simulink model "Der_Faux_FPGA_V2_optimized_synthesizable"  (R2020a)
settings: Solver=FixedStepDiscrete  StartTime=0.0  StopTime=0.84375  FixedStep=1/fs_sim  RelTol=1e-3
values from neighbouring files (symbols this model uses):
  ADC_res = 5    [Der_Faux_ctr_FPGA.m]
  ADC_res_G4 = 8    [Der_Faux_ctr_FPGA.m]
  fs = 48000    [Der_Faux_ctr_FPGA.m]
  fs_sim = fs*ovs    (= 6144000)    [Der_Faux_ctr_FPGA.m]
  Gvar1_N = fi(Gvar1_N,0,ADC_res,0)    [Der_Faux_ctr_FPGA.m]
  Gvar2_N = fi(Gvar2_N,0,ADC_res,0)    [Der_Faux_ctr_FPGA.m]
  Gvar3_N = fi(Gvar3_N,0,ADC_res,0)    [Der_Faux_ctr_FPGA.m]
  Gvar4_N = fi(Gvar4_N,0,ADC_res_G4,0)    [Der_Faux_ctr_FPGA.m]
  input_space = linspace(0,2^ADC_res-1,2^ADC_res)    [Der_Faux_ctr_FPGA.m]
  input_spcae_extended = linspace(0,(2^ADC_res)^3-1,(2^ADC_res)^3)    [Der_Faux_ctr_FPGA.m]
  LUT_Z22a_opt = sfi(LUT_Z22a, len_LUT22a)    [Der_Faux_ctr_FPGA.m]
  LUT_Z22b_opt = sfi(LUT_Z22b, len_LUT22b)    [Der_Faux_ctr_FPGA.m]
  LUT_Z23a_opt = sfi(LUT_Z23a, len_Z23a)    [Der_Faux_ctr_FPGA.m]
  LUT_Z23b_opt = sfi(LUT_Z23b, len_Z23b)    [Der_Faux_ctr_FPGA.m]
  LUT_Z24a_opt = sfi(LUT_Z24a, len_LUT24a)    [Der_Faux_ctr_FPGA.m]
  LUT_Z24b_opt = sfi(LUT_Z24b, len_LUT24b)    [Der_Faux_ctr_FPGA.m]
  LUT_Z25a_opt = sfi(LUT_Z25a, len_LUT25a)    [Der_Faux_ctr_FPGA.m]
  LUT_Z25b_opt = sfi(LUT_Z25b, len_LUT25b)    [Der_Faux_ctr_FPGA.m]
  shift_reg_size = 8*44000    (= 352000)    [Der_Faux_ctr_FPGA.m]
  use_stimuli = [true,true,true,true]    [Der_Faux_ctr_FPGA.m]
  WL_RAM = 5    [Der_Faux_ctr_FPGA.m]
undefined symbols (not defined in the file or in its folder): poti_stimuli1, poti_stimuli2, poti_stimuli3, poti_stimuli4
libraries: hdlmdlgenlib x30, simulink x6, hdlsllib x4
(part 3 of 3)

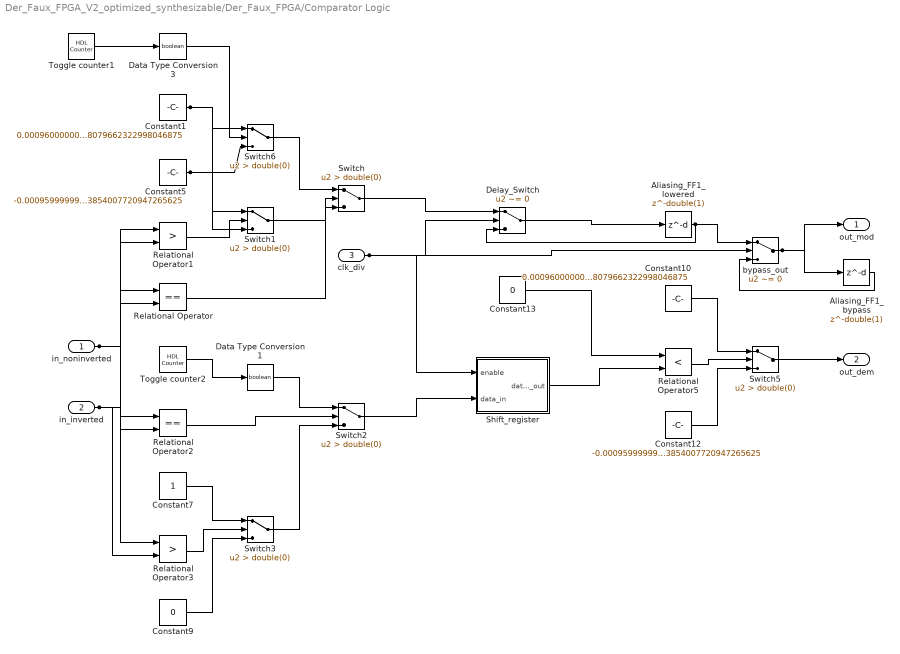
== system Der_Faux_FPGA_V2_optimized_synthesizable/Der_Faux_FPGA/Comparator Logic ==
  in_noninverted : Inport  OutDataTypeStr=fixdt(1, 46, 42)  PortDimensions=1  SampleTime=1.62760416666667e-07
  in_inverted : Inport  Port=2  OutDataTypeStr=fixdt(1, 46, 42)  PortDimensions=1  SampleTime=1.62760416666667e-07
  clk_div : Inport  Port=3  OutDataTypeStr=boolean  PortDimensions=1  SampleTime=1.62760416666667e-07  LockScale=on
  Aliasing_FF1_bypass : Delay  DelayLength=double(1)  SampleTime=1.62760416666667e-07
  Aliasing_FF1_lowered : Delay  DelayLength=double(1)  InitialCondition=0  SampleTime=1.62760416666667e-07
  Constant1 : Constant  Value=0.00096000000000000251798581984985503368079662322998046875  OutDataTypeStr=fixdt(0, 46, 56)  SampleTime=1.62760416666667e-07
  Constant10 : Constant  Value=0.00096000000000000251798581984985503368079662322998046875  OutDataTypeStr=fixdt(0, 46, 56)  SampleTime=1.62760416666667e-07
  Constant12 : Constant  Value=-0.0009599999999999886401980120353982783854007720947265625  OutDataTypeStr=fixdt(1, 46, 55)  SampleTime=1.62760416666667e-07
  Constant13 : Constant  Value=0  OutDataTypeStr=boolean  SampleTime=1.62760416666667e-07
  Constant5 : Constant  Value=-0.0009599999999999886401980120353982783854007720947265625  OutDataTypeStr=fixdt(1, 46, 55)  SampleTime=1.62760416666667e-07
  Constant7 : Constant  OutDataTypeStr=boolean  SampleTime=1.62760416666667e-07
  Constant9 : Constant  Value=0  OutDataTypeStr=boolean  SampleTime=1.62760416666667e-07
  Data Type Conversion1 : DataTypeConversion  OutDataTypeStr=boolean  SampleTime=1.62760416666667e-07
  Data Type Conversion3 : DataTypeConversion  OutDataTypeStr=boolean  SampleTime=1.62760416666667e-07
  Delay_Switch : Switch  Criteria=u2 ~= 0  Threshold=double(0)  OutDataTypeStr=fixdt(1, 46, 54)  SampleTime=1.62760416666667e-07
  Relational Operator : RelationalOperator  Operator===  OutDataTypeStr=boolean  SampleTime=1.62760416666667e-07  RndMeth=Nearest
  Relational Operator1 : RelationalOperator  Operator=>  OutDataTypeStr=boolean  SampleTime=1.62760416666667e-07  RndMeth=Nearest
  Relational Operator2 : RelationalOperator  Operator===  OutDataTypeStr=boolean  SampleTime=1.62760416666667e-07  RndMeth=Nearest
  Relational Operator3 : RelationalOperator  Operator=>  OutDataTypeStr=boolean  SampleTime=1.62760416666667e-07  RndMeth=Nearest
  Relational Operator5 : RelationalOperator  Operator=<  OutDataTypeStr=boolean  SampleTime=1.62760416666667e-07  RndMeth=Nearest
  Shift_register : Subsystem
  Switch{,1,5..6} (4 alike) : Switch  Criteria=u2 > Threshold  Threshold=double(0)  OutDataTypeStr=fixdt(1, 46, 54)  SampleTime=1.62760416666667e-07
  Switch2 : Switch  Criteria=u2 > Threshold  Threshold=double(0)  OutDataTypeStr=boolean  SampleTime=1.62760416666667e-07
  Switch3 : Switch  Criteria=u2 > Threshold  Threshold=double(0)  OutDataTypeStr=boolean  SampleTime=1.62760416666667e-07
  Toggle counter1 : hdlsllib/Sources/HDL Counter  CountType=Count limited  CountInit=double(0)  CountStep=double(1)  CountMax=double(1)  CountFromType=Initial value  CountFrom=double(0)  CountResetPort=off  CountLoadPort=off  CountEnbPort=off  CountDirPort=off  CountDataType=Unsigned  CountWordLen=1  CountFracLen=0  CountSampTime=1.62760416666667e-07
  Toggle counter2 : hdlsllib/Sources/HDL Counter  CountType=Count limited  CountInit=double(0)  CountStep=double(1)  CountMax=double(1)  CountFromType=Initial value  CountFrom=double(0)  CountResetPort=off  CountLoadPort=off  CountEnbPort=off  CountDirPort=off  CountDataType=Unsigned  CountWordLen=1  CountFracLen=0  CountSampTime=1.62760416666667e-07
  bypass_out : Switch  Criteria=u2 ~= 0  Threshold=double(0)  OutDataTypeStr=fixdt(1, 46, 54)  SampleTime=1.62760416666667e-07
  out_mod : Outport  OutDataTypeStr=fixdt(1,46,54)  SampleTime=1/fs_sim
  out_dem : Outport  Port=2  OutDataTypeStr=fixdt(1,46,54)  SampleTime=1/fs_sim
  wires:
  in_noninverted/1 -> Relational Operator3/1, Relational Operator2/1, Relational Operator1/1, Relational Operator/1
  in_inverted/1 -> Relational Operator3/2, Relational Operator2/2, Relational Operator1/2, Relational Operator/2
  clk_div/1 -> bypass_out/2, Delay_Switch/2, Shift_register/1(enable)
  bypass_out/1 -> Aliasing_FF1_bypass/1, out_mod/1
  Constant1/1 -> Switch6/1, Switch1/1
  Constant10/1 -> Switch5/1
  Constant12/1 -> Switch5/3
  Constant13/1 -> Relational Operator5/1
  Constant5/1 -> Switch6/3, Switch1/3
  Constant7/1 -> Switch3/1
  Constant9/1 -> Switch3/3
  Data Type Conversion1/1 -> Switch2/1
  Data Type Conversion3/1 -> Switch6/2
  Relational Operator/1 -> Switch/2
  Relational Operator1/1 -> Switch1/2
  Relational Operator2/1 -> Switch2/2
  Relational Operator3/1 -> Switch3/2
  Relational Operator5/1 -> Switch5/2
  Shift_register/1(data_out) -> Relational Operator5/2
  Switch/1 -> Delay_Switch/1
  Switch1/1 -> Switch/3
  Switch2/1 -> Shift_register/2(data_in)
  Switch3/1 -> Switch2/3
  Switch5/1 -> out_dem/1
  Switch6/1 -> Switch/1
  Toggle counter1/1 -> Data Type Conversion3/1
  Toggle counter2/1 -> Data Type Conversion1/1
  Aliasing_FF1_lowered/1 -> bypass_out/1, Delay_Switch/3
  Delay_Switch/1 -> Aliasing_FF1_lowered/1
  Aliasing_FF1_bypass/1 -> bypass_out/3

== system Der_Faux_FPGA_V2_optimized_synthesizable/Der_Faux_FPGA/Difference1 ==
  note: U(k)
  note: ( U(k) - U(k-1) )
  U : Inport  OutDataTypeStr=fixdt(1, 46, 76)  SampleTime=1.62760416666667e-07
  Diff : Sum  Description=Add in CPU  Inputs=+-  OutMin=OutMin  OutMax=OutMax  OutDataTypeStr=OutDataTypeStr  SaturateOnIntegerOverflow=on
  UD : UnitDelay  Description=Store in Global RAM  DisableCoverage=on  InitialCondition=ICPrevInput  SampleTime=-1  HasFrameUpgradeWarning=on
  Y : Outport
  wires:
  U/1 -> Diff/1, UD/1
  Diff/1 -> Y/1
  UD/1 -> Diff/2

== system Der_Faux_FPGA_V2_optimized_synthesizable/Der_Faux_FPGA/Difference10 ==
  note: U(k)
  note: ( U(k) - U(k-1) )
  U : Inport  OutDataTypeStr=fixdt(1, 46, 66)  SampleTime=1.62760416666667e-07
  Diff : Sum  Description=Add in CPU  Inputs=+-  OutMin=OutMin  OutMax=OutMax  OutDataTypeStr=OutDataTypeStr  SaturateOnIntegerOverflow=on
  UD : UnitDelay  Description=Store in Global RAM  DisableCoverage=on  InitialCondition=ICPrevInput  SampleTime=-1  HasFrameUpgradeWarning=on
  Y : Outport
  wires:
  U/1 -> Diff/1, UD/1
  Diff/1 -> Y/1
  UD/1 -> Diff/2

== system Der_Faux_FPGA_V2_optimized_synthesizable/Der_Faux_FPGA/Difference11 ==
  note: U(k)
  note: ( U(k) - U(k-1) )
  U : Inport  OutDataTypeStr=fixdt(1, 46, 66)  SampleTime=1.62760416666667e-07
  Diff : Sum  Description=Add in CPU  Inputs=+-  OutMin=OutMin  OutMax=OutMax  OutDataTypeStr=OutDataTypeStr  SaturateOnIntegerOverflow=on
  UD : UnitDelay  Description=Store in Global RAM  DisableCoverage=on  InitialCondition=ICPrevInput  SampleTime=-1  HasFrameUpgradeWarning=on
  Y : Outport
  wires:
  U/1 -> Diff/1, UD/1
  Diff/1 -> Y/1
  UD/1 -> Diff/2

== system Der_Faux_FPGA_V2_optimized_synthesizable/Der_Faux_FPGA/Difference12 ==
  note: U(k)
  note: ( U(k) - U(k-1) )
  U : Inport  OutDataTypeStr=fixdt(1, 46, 62)  SampleTime=1.62760416666667e-07
  Diff : Sum  Description=Add in CPU  Inputs=+-  OutMin=OutMin  OutMax=OutMax  OutDataTypeStr=OutDataTypeStr  SaturateOnIntegerOverflow=on
  UD : UnitDelay  Description=Store in Global RAM  DisableCoverage=on  InitialCondition=ICPrevInput  SampleTime=-1  HasFrameUpgradeWarning=on
  Y : Outport
  wires:
  U/1 -> Diff/1, UD/1
  Diff/1 -> Y/1
  UD/1 -> Diff/2

== system Der_Faux_FPGA_V2_optimized_synthesizable/Der_Faux_FPGA/Difference13 ==
  note: U(k)
  note: ( U(k) - U(k-1) )
  U : Inport  OutDataTypeStr=fixdt(1, 46, 63)  SampleTime=1.62760416666667e-07
  Diff : Sum  Description=Add in CPU  Inputs=+-  OutMin=OutMin  OutMax=OutMax  OutDataTypeStr=OutDataTypeStr  SaturateOnIntegerOverflow=on
  UD : UnitDelay  Description=Store in Global RAM  DisableCoverage=on  InitialCondition=ICPrevInput  SampleTime=-1  HasFrameUpgradeWarning=on
  Y : Outport
  wires:
  U/1 -> Diff/1, UD/1
  Diff/1 -> Y/1
  UD/1 -> Diff/2

== system Der_Faux_FPGA_V2_optimized_synthesizable/Der_Faux_FPGA/Difference3 ==
  note: U(k)
  note: ( U(k) - U(k-1) )
  U : Inport  OutDataTypeStr=fixdt(1, 46, 43)  SampleTime=1.62760416666667e-07
  Diff : Sum  Description=Add in CPU  Inputs=+-  OutMin=OutMin  OutMax=OutMax  OutDataTypeStr=OutDataTypeStr  SaturateOnIntegerOverflow=on
  UD : UnitDelay  Description=Store in Global RAM  DisableCoverage=on  InitialCondition=ICPrevInput  SampleTime=-1  HasFrameUpgradeWarning=on
  Y : Outport
  wires:
  U/1 -> Diff/1, UD/1
  Diff/1 -> Y/1
  UD/1 -> Diff/2

== system Der_Faux_FPGA_V2_optimized_synthesizable/Der_Faux_FPGA/Difference4 ==
  note: U(k)
  note: ( U(k) - U(k-1) )
  U : Inport  OutDataTypeStr=fixdt(1, 46, 73)  SampleTime=1.62760416666667e-07
  Diff : Sum  Description=Add in CPU  Inputs=+-  OutMin=OutMin  OutMax=OutMax  OutDataTypeStr=OutDataTypeStr  SaturateOnIntegerOverflow=on
  UD : UnitDelay  Description=Store in Global RAM  DisableCoverage=on  InitialCondition=ICPrevInput  SampleTime=-1  HasFrameUpgradeWarning=on
  Y : Outport
  wires:
  U/1 -> Diff/1, UD/1
  Diff/1 -> Y/1
  UD/1 -> Diff/2

== system Der_Faux_FPGA_V2_optimized_synthesizable/Der_Faux_FPGA/Difference5 ==
  note: U(k)
  note: ( U(k) - U(k-1) )
  U : Inport  OutDataTypeStr=fixdt(1, 46, 66)  SampleTime=1.62760416666667e-07
  Diff : Sum  Description=Add in CPU  Inputs=+-  OutMin=OutMin  OutMax=OutMax  OutDataTypeStr=OutDataTypeStr  SaturateOnIntegerOverflow=on
  UD : UnitDelay  Description=Store in Global RAM  DisableCoverage=on  InitialCondition=ICPrevInput  SampleTime=-1  HasFrameUpgradeWarning=on
  Y : Outport
  wires:
  U/1 -> Diff/1, UD/1
  Diff/1 -> Y/1
  UD/1 -> Diff/2

== system Der_Faux_FPGA_V2_optimized_synthesizable/Der_Faux_FPGA/Difference6 ==
  note: U(k)
  note: ( U(k) - U(k-1) )
  U : Inport  OutDataTypeStr=fixdt(1, 46, 65)  SampleTime=1.62760416666667e-07
  Diff : Sum  Description=Add in CPU  Inputs=+-  OutMin=OutMin  OutMax=OutMax  OutDataTypeStr=OutDataTypeStr  SaturateOnIntegerOverflow=on
  UD : UnitDelay  Description=Store in Global RAM  DisableCoverage=on  InitialCondition=ICPrevInput  SampleTime=-1  HasFrameUpgradeWarning=on
  Y : Outport
  wires:
  U/1 -> Diff/1, UD/1
  Diff/1 -> Y/1
  UD/1 -> Diff/2

== system Der_Faux_FPGA_V2_optimized_synthesizable/Der_Faux_FPGA/Difference7 ==
  note: U(k)
  note: ( U(k) - U(k-1) )
  U : Inport  OutDataTypeStr=fixdt(1, 46, 73)  SampleTime=1.62760416666667e-07
  Diff : Sum  Description=Add in CPU  Inputs=+-  OutMin=OutMin  OutMax=OutMax  OutDataTypeStr=OutDataTypeStr  SaturateOnIntegerOverflow=on
  UD : UnitDelay  Description=Store in Global RAM  DisableCoverage=on  InitialCondition=ICPrevInput  SampleTime=-1  HasFrameUpgradeWarning=on
  Y : Outport
  wires:
  U/1 -> Diff/1, UD/1
  Diff/1 -> Y/1
  UD/1 -> Diff/2

== system Der_Faux_FPGA_V2_optimized_synthesizable/Der_Faux_FPGA/Difference8 ==
  note: U(k)
  note: ( U(k) - U(k-1) )
  U : Inport  OutDataTypeStr=fixdt(1, 46, 63)  SampleTime=1.62760416666667e-07
  Diff : Sum  Description=Add in CPU  Inputs=+-  OutMin=OutMin  OutMax=OutMax  OutDataTypeStr=OutDataTypeStr  SaturateOnIntegerOverflow=on
  UD : UnitDelay  Description=Store in Global RAM  DisableCoverage=on  InitialCondition=ICPrevInput  SampleTime=-1  HasFrameUpgradeWarning=on
  Y : Outport
  wires:
  U/1 -> Diff/1, UD/1
  Diff/1 -> Y/1
  UD/1 -> Diff/2

== system Der_Faux_FPGA_V2_optimized_synthesizable/Der_Faux_FPGA/Difference9 ==
  note: U(k)
  note: ( U(k) - U(k-1) )
  U : Inport  OutDataTypeStr=fixdt(1, 46, 62)  SampleTime=1.62760416666667e-07
  Diff : Sum  Description=Add in CPU  Inputs=+-  OutMin=OutMin  OutMax=OutMax  OutDataTypeStr=OutDataTypeStr  SaturateOnIntegerOverflow=on
  UD : UnitDelay  Description=Store in Global RAM  DisableCoverage=on  InitialCondition=ICPrevInput  SampleTime=-1  HasFrameUpgradeWarning=on
  Y : Outport
  wires:
  U/1 -> Diff/1, UD/1
  Diff/1 -> Y/1
  UD/1 -> Diff/2

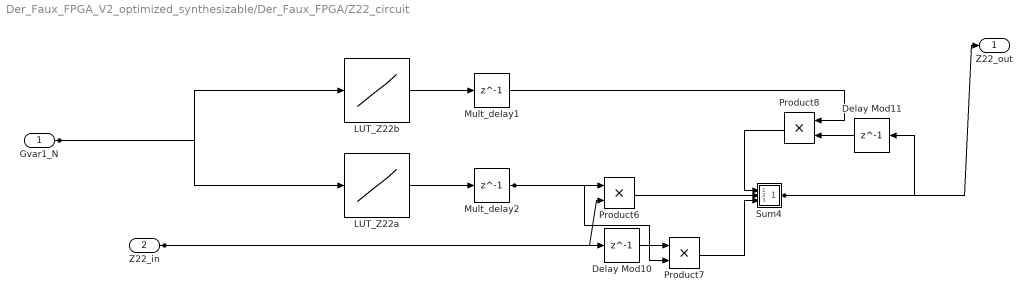
== system Der_Faux_FPGA_V2_optimized_synthesizable/Der_Faux_FPGA/Z22_circuit ==
  Gvar1_N : Inport  OutDataTypeStr=fixdt(0, 5, 0)  PortDimensions=1  SampleTime=1.62760416666667e-07  LockScale=on
  Z22_in : Inport  Port=2  OutDataTypeStr=fixdt(1, 46, 52)  PortDimensions=1  SampleTime=1.62760416666667e-07
  Delay Mod10 : Delay  DelayLength=1  InitialCondition=0  SampleTime=1/fs_sim
  Delay Mod11 : Delay  DelayLength=1  InitialCondition=0  SampleTime=1/fs_sim
  LUT_Z22a : Lookup_n-D  NumberOfTableDimensions=1  LookupTableObject=''  BreakpointsForDimension1=input_space  BreakpointsForDimension1FirstPoint=10  BreakpointsForDimension2FirstPoint=10  BreakpointsForDimension1Spacing=12  BreakpointsForDimension2Spacing=12  BreakpointsForDimension1DataTypeStr=Inherit: Inherit from 'Breakpoint data'  IndexSearchMethod=Evenly spaced points  Table=LUT_Z22a_opt  TableDataTypeStr=Inherit: Inherit from 'Table data'  InterpMethod=Flat  DiagnosticForOutOfRangeInput=Error  InternalRulePriority=Speed  OutDataTypeStr=Inherit: Inherit from 'Table data'  RndMeth=Simplest  InputSameDT=on  LockScale=on
  LUT_Z22b : Lookup_n-D  NumberOfTableDimensions=1  LookupTableObject=''  BreakpointsForDimension1=input_space  BreakpointsForDimension1FirstPoint=10  BreakpointsForDimension2FirstPoint=10  BreakpointsForDimension1Spacing=12  BreakpointsForDimension2Spacing=12  BreakpointsForDimension1DataTypeStr=Inherit: Inherit from 'Breakpoint data'  IndexSearchMethod=Evenly spaced points  Table=LUT_Z22b_opt  TableDataTypeStr=Inherit: Inherit from 'Table data'  InterpMethod=Flat  DiagnosticForOutOfRangeInput=Error  InternalRulePriority=Speed  OutDataTypeStr=Inherit: Inherit from 'Table data'  RndMeth=Simplest  InputSameDT=on  LockScale=on
  Mult_delay1 : Delay  DelayLength=1
  Mult_delay2 : Delay  DelayLength=1
  Product6 : Product  OutDataTypeStr=fixdt(1,46,53)  SaturateOnIntegerOverflow=on
  Product7 : Product  OutDataTypeStr=fixdt(1,46,53)  SaturateOnIntegerOverflow=on
  Product8 : Product  OutDataTypeStr=fixdt(1,46,43)  SaturateOnIntegerOverflow=on
  Sum4 : Subsystem
  Z22_out : Outport
  wires:
  Gvar1_N/1 -> LUT_Z22b/1, LUT_Z22a/1
  Z22_in/1 -> Product6/2, Delay Mod10/1
  Delay Mod10/1 -> Product7/1
  Delay Mod11/1 -> Product8/2
  LUT_Z22a/1 -> Mult_delay2/1
  LUT_Z22b/1 -> Mult_delay1/1
  Mult_delay1/1 -> Product8/1
  Mult_delay2/1 -> Product7/2, Product6/1
  Product6/1 -> Sum4/2(In2)
  Product7/1 -> Sum4/3(In3)
  Product8/1 -> Sum4/1(In1)
  Sum4/1(Out1) -> Delay Mod11/1, Z22_out/1

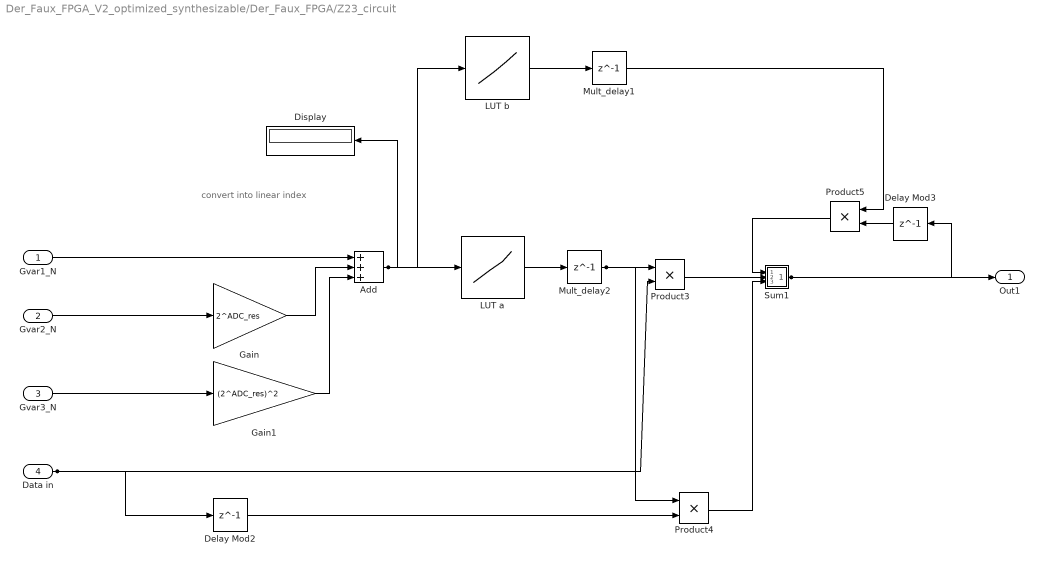
== system Der_Faux_FPGA_V2_optimized_synthesizable/Der_Faux_FPGA/Z23_circuit ==
  note: convert into linear index
  Gvar1_N : Inport  OutDataTypeStr=fixdt(0, 5, 0)  PortDimensions=1  SampleTime=1.62760416666667e-07  LockScale=on
  Gvar2_N : Inport  Port=2  OutDataTypeStr=fixdt(0, 5, 0)  PortDimensions=1  SampleTime=1.62760416666667e-07  LockScale=on
  Gvar3_N : Inport  Port=3  OutDataTypeStr=fixdt(0, 5, 0)  PortDimensions=1  SampleTime=1.62760416666667e-07  LockScale=on
  Data in : Inport  Port=4  OutDataTypeStr=fixdt(1, 46, 50)  PortDimensions=1  SampleTime=1.62760416666667e-07  LockScale=on
  Add : Sum  Inputs=+++  AccumDataTypeStr=fixdt(0,N_ext,0)  LockScale=on
  Delay Mod2 : Delay  DelayLength=1  InitialCondition=0  SampleTime=1/fs_sim
  Delay Mod3 : Delay  DelayLength=1  InitialCondition=0  SampleTime=1/fs_sim
  Display : Display
  Gain : Gain  Gain=2^ADC_res  OutDataTypeStr=fixdt(0,N_ext,0)  LockScale=on
  Gain1 : Gain  Gain=(2^ADC_res)^2  OutDataTypeStr=fixdt(0,N_ext,0)  LockScale=on
  "LUT a " : Lookup_n-D  NumberOfTableDimensions=1  LookupTableObject=''  BreakpointsForDimension1=input_spcae_extended  BreakpointsForDimension2=0:3  BreakpointsForDimension3=0:3  BreakpointsForDimension1FirstPoint=10  BreakpointsForDimension2FirstPoint=10  BreakpointsForDimension1Spacing=12  BreakpointsForDimension2Spacing=12  BreakpointsForDimension1DataTypeStr=Inherit: Inherit from 'Breakpoint data'  BreakpointsForDimension2DataTypeStr=Inherit: Inherit from 'Breakpoint data'  BreakpointsForDimension3DataTypeStr=Inherit: Inherit from 'Breakpoint data'  IndexSearchMethod=Evenly spaced points  Table=LUT_Z23a_opt  TableDataTypeStr=Inherit: Inherit from 'Table data'  InterpMethod=Flat  DiagnosticForOutOfRangeInput=Error  InternalRulePriority=Speed  OutDataTypeStr=Inherit: Inherit from 'Table data'  RndMeth=Simplest  InputSameDT=on  LockScale=on
  LUT b : Lookup_n-D  NumberOfTableDimensions=1  LookupTableObject=''  BreakpointsForDimension1=input_spcae_extended  BreakpointsForDimension2=0:3  BreakpointsForDimension3=0:3  BreakpointsForDimension1FirstPoint=10  BreakpointsForDimension2FirstPoint=10  BreakpointsForDimension1Spacing=12  BreakpointsForDimension2Spacing=12  BreakpointsForDimension1DataTypeStr=Inherit: Inherit from 'Breakpoint data'  BreakpointsForDimension2DataTypeStr=Inherit: Inherit from 'Breakpoint data'  BreakpointsForDimension3DataTypeStr=Inherit: Inherit from 'Breakpoint data'  IndexSearchMethod=Evenly spaced points  Table=LUT_Z23b_opt  TableDataTypeStr=Inherit: Inherit from 'Table data'  InterpMethod=Flat  DiagnosticForOutOfRangeInput=Error  InternalRulePriority=Speed  OutDataTypeStr=Inherit: Inherit from 'Table data'  RndMeth=Simplest  InputSameDT=on  LockScale=on
  Mult_delay1 : Delay  DelayLength=1
  Mult_delay2 : Delay  DelayLength=1
  Product3 : Product  OutDataTypeStr=fixdt(1,46,54)  SaturateOnIntegerOverflow=on
  Product4 : Product  OutDataTypeStr=fixdt(1,46,54)  SaturateOnIntegerOverflow=on
  Product5 : Product  OutDataTypeStr=fixdt(1,46,42)  SaturateOnIntegerOverflow=on
  Sum1 : Subsystem
  Out1 : Outport
  wires:
  Gvar1_N/1 -> Add/1
  Gvar2_N/1 -> Gain/1
  Gvar3_N/1 -> Gain1/1
  Data in/1 -> Product3/2, Delay Mod2/1
  Add/1 -> LUT b/1, "LUT a "/1, Display/1
  Delay Mod2/1 -> Product4/2
  Delay Mod3/1 -> Product5/2
  Gain/1 -> Add/2
  Gain1/1 -> Add/3
  "LUT a "/1 -> Mult_delay2/1
  LUT b/1 -> Mult_delay1/1
  Mult_delay1/1 -> Product5/1
  Mult_delay2/1 -> Product4/1, Product3/1
  Product3/1 -> Sum1/2(In2)
  Product4/1 -> Sum1/3(In3)
  Product5/1 -> Sum1/1(In1)
  Sum1/1(Out1) -> Delay Mod3/1, Out1/1

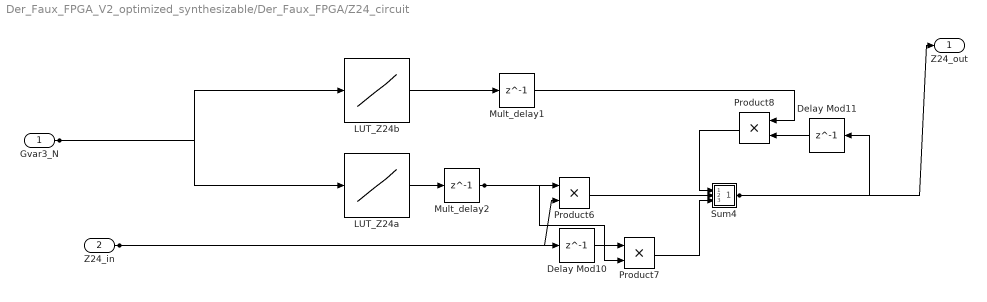
== system Der_Faux_FPGA_V2_optimized_synthesizable/Der_Faux_FPGA/Z24_circuit ==
  Gvar3_N : Inport  OutDataTypeStr=fixdt(0, 5, 0)  PortDimensions=1  SampleTime=1.62760416666667e-07  LockScale=on
  Z24_in : Inport  Port=2  OutDataTypeStr=fixdt(1, 46, 51)  PortDimensions=1  SampleTime=1.62760416666667e-07
  Delay Mod10 : Delay  DelayLength=1  InitialCondition=0  SampleTime=1/fs_sim
  Delay Mod11 : Delay  DelayLength=1  InitialCondition=0  SampleTime=1/fs_sim
  LUT_Z24a : Lookup_n-D  NumberOfTableDimensions=1  LookupTableObject=''  BreakpointsForDimension1=input_space  BreakpointsForDimension1FirstPoint=10  BreakpointsForDimension2FirstPoint=10  BreakpointsForDimension1Spacing=12  BreakpointsForDimension2Spacing=12  BreakpointsForDimension1DataTypeStr=Inherit: Inherit from 'Breakpoint data'  IndexSearchMethod=Evenly spaced points  Table=LUT_Z24a_opt  TableDataTypeStr=Inherit: Inherit from 'Table data'  InterpMethod=Flat  DiagnosticForOutOfRangeInput=Error  InternalRulePriority=Speed  OutDataTypeStr=Inherit: Inherit from 'Table data'  RndMeth=Simplest  InputSameDT=on  LockScale=on
  LUT_Z24b : Lookup_n-D  NumberOfTableDimensions=1  LookupTableObject=''  BreakpointsForDimension1=input_space  BreakpointsForDimension1FirstPoint=10  BreakpointsForDimension2FirstPoint=10  BreakpointsForDimension1Spacing=12  BreakpointsForDimension2Spacing=12  BreakpointsForDimension1DataTypeStr=Inherit: Inherit from 'Breakpoint data'  IndexSearchMethod=Evenly spaced points  Table=LUT_Z24b_opt  TableDataTypeStr=Inherit: Inherit from 'Table data'  InterpMethod=Flat  DiagnosticForOutOfRangeInput=Error  InternalRulePriority=Speed  OutDataTypeStr=Inherit: Inherit from 'Table data'  RndMeth=Simplest  InputSameDT=on  LockScale=on
  Mult_delay1 : Delay  DelayLength=1
  Mult_delay2 : Delay  DelayLength=1
  Product6 : Product  OutDataTypeStr=fixdt(1,46,54)  SaturateOnIntegerOverflow=on
  Product7 : Product  OutDataTypeStr=fixdt(1,46,54)  SaturateOnIntegerOverflow=on
  Product8 : Product  OutDataTypeStr=fixdt(1,46,43)  SaturateOnIntegerOverflow=on
  Sum4 : Subsystem
  Z24_out : Outport
  wires:
  Gvar3_N/1 -> LUT_Z24b/1, LUT_Z24a/1
  Z24_in/1 -> Product6/2, Delay Mod10/1
  Delay Mod10/1 -> Product7/1
  Delay Mod11/1 -> Product8/2
  LUT_Z24a/1 -> Mult_delay2/1
  LUT_Z24b/1 -> Mult_delay1/1
  Mult_delay1/1 -> Product8/1
  Mult_delay2/1 -> Product7/2, Product6/1
  Product6/1 -> Sum4/2(In2)
  Product7/1 -> Sum4/3(In3)
  Product8/1 -> Sum4/1(In1)
  Sum4/1(Out1) -> Delay Mod11/1, Z24_out/1

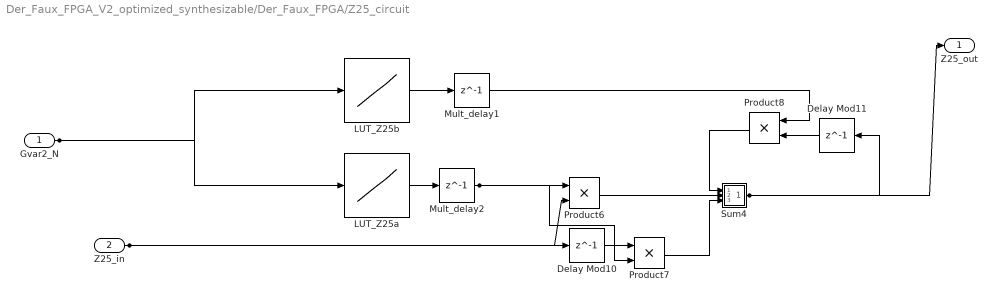
== system Der_Faux_FPGA_V2_optimized_synthesizable/Der_Faux_FPGA/Z25_circuit ==
  Gvar2_N : Inport  OutDataTypeStr=fixdt(0, 5, 0)  PortDimensions=1  SampleTime=1.62760416666667e-07  LockScale=on
  Z25_in : Inport  Port=2  OutDataTypeStr=fixdt(1, 46, 51)  PortDimensions=1  SampleTime=1.62760416666667e-07
  Delay Mod10 : Delay  DelayLength=1  InitialCondition=0  SampleTime=1/fs_sim
  Delay Mod11 : Delay  DelayLength=1  InitialCondition=0  SampleTime=1/fs_sim
  LUT_Z25a : Lookup_n-D  NumberOfTableDimensions=1  LookupTableObject=''  BreakpointsForDimension1=input_space  BreakpointsForDimension1FirstPoint=10  BreakpointsForDimension2FirstPoint=10  BreakpointsForDimension1Spacing=12  BreakpointsForDimension2Spacing=12  IndexSearchMethod=Evenly spaced points  Table=LUT_Z25a_opt  TableDataTypeStr=Inherit: Inherit from 'Table data'  InterpMethod=Flat  DiagnosticForOutOfRangeInput=Error  InternalRulePriority=Speed  OutDataTypeStr=Inherit: Inherit from 'Table data'  RndMeth=Simplest  InputSameDT=on  LockScale=on
  LUT_Z25b : Lookup_n-D  NumberOfTableDimensions=1  LookupTableObject=''  BreakpointsForDimension1=input_space  BreakpointsForDimension1FirstPoint=10  BreakpointsForDimension2FirstPoint=10  BreakpointsForDimension1Spacing=12  BreakpointsForDimension2Spacing=12  IndexSearchMethod=Evenly spaced points  Table=LUT_Z25b_opt  TableDataTypeStr=Inherit: Inherit from 'Table data'  InterpMethod=Flat  DiagnosticForOutOfRangeInput=Error  InternalRulePriority=Speed  OutDataTypeStr=Inherit: Inherit from 'Table data'  RndMeth=Simplest  InputSameDT=on  LockScale=on
  Mult_delay1 : Delay  DelayLength=1
  Mult_delay2 : Delay  DelayLength=1
  Product6 : Product  OutDataTypeStr=fixdt(1,46,50)  SaturateOnIntegerOverflow=on
  Product7 : Product  OutDataTypeStr=fixdt(1,46,50)  SaturateOnIntegerOverflow=on
  Product8 : Product  OutDataTypeStr=fixdt(1,46,42)  SaturateOnIntegerOverflow=on
  Sum4 : Subsystem
  Z25_out : Outport
  wires:
  Gvar2_N/1 -> LUT_Z25b/1, LUT_Z25a/1
  Z25_in/1 -> Product6/2, Delay Mod10/1
  Delay Mod10/1 -> Product7/1
  Delay Mod11/1 -> Product8/2
  LUT_Z25a/1 -> Mult_delay2/1
  LUT_Z25b/1 -> Mult_delay1/1
  Mult_delay1/1 -> Product8/1
  Mult_delay2/1 -> Product7/2, Product6/1
  Product6/1 -> Sum4/2(In2)
  Product7/1 -> Sum4/3(In3)
  Product8/1 -> Sum4/1(In1)
  Sum4/1(Out1) -> Delay Mod11/1, Z25_out/1

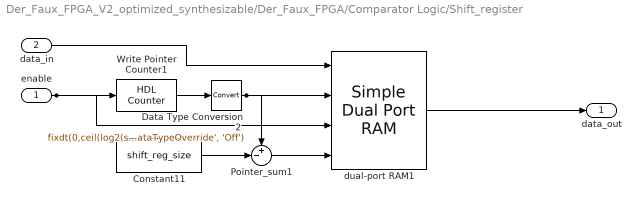
== system Der_Faux_FPGA_V2_optimized_synthesizable/Der_Faux_FPGA/Comparator Logic/Shift_register ==
  enable : Inport  OutDataTypeStr=boolean  PortDimensions=1  SampleTime=1.62760416666667e-07
  data_in : Inport  Port=2  OutDataTypeStr=boolean  PortDimensions=1  SampleTime=1.62760416666667e-07
  Constant11 : Constant  Value=shift_reg_size  OutDataTypeStr=fixdt(0,ceil(log2(shift_reg_size)),0, 'DataTypeOverride', 'Off')  SampleTime=1/(fs_sim)  LockScale=on
  Data Type Conversion2 : DataTypeConversion  OutDataTypeStr=fixdt(0,ceil(log2(shift_reg_size)),0, 'DataTypeOverride', 'Off')  LockScale=on
  Pointer_sum1 : Sum  Inputs=+-|  OutDataTypeStr=fixdt(0,ceil(log2(shift_reg_size)),0, 'DataTypeOverride', 'Off')  LockScale=on
  Write Pointer Counter1 : hdlsllib/Sources/HDL Counter  CountType=Count limited  CountInit=0  CountStep=1  CountMax=2^ceil(log2(shift_reg_size))-1  CountFromType=Initial value  CountFrom=0  CountResetPort=off  CountLoadPort=off  CountEnbPort=on  CountDirPort=off  CountDataType=Unsigned  CountWordLen=ceil(log2(shift_reg_size))  CountFracLen=0  CountSampTime=1/(fs_sim/WL_RAM)
  dual-port RAM1 : hdlsllib/HDL RAMs/Simple Dual Port RAM  ram_size=ceil(log2(shift_reg_size))
      settings: SourceProductBaseCode=SL
  data_out : Outport
  wires:
  enable/1 -> Write Pointer Counter1/1, dual-port RAM1/3
  data_in/1 -> dual-port RAM1/1
  Constant11/1 -> Pointer_sum1/2
  Data Type Conversion2/1 -> Pointer_sum1/1, dual-port RAM1/2
  Pointer_sum1/1 -> dual-port RAM1/4
  Write Pointer Counter1/1 -> Data Type Conversion2/1
  dual-port RAM1/1 -> data_out/1

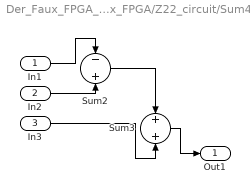
== system Der_Faux_FPGA_V2_optimized_synthesizable/Der_Faux_FPGA/Z22_circuit/Sum4 ==
  In1 : Inport  OutDataTypeStr=fixdt(1,46,43)
  In2 : Inport  Port=2  OutDataTypeStr=fixdt(1,46,53)
  In3 : Inport  Port=3  OutDataTypeStr=fixdt(1,46,53)
  Sum2 : Sum  Inputs=-+  AccumDataTypeStr=fixdt(1,57,53)  OutDataTypeStr=fixdt(1,57,53)  SaturateOnIntegerOverflow=on
  Sum3 : Sum  AccumDataTypeStr=fixdt(1,57,53)  OutDataTypeStr=fixdt(1,46,43)  SaturateOnIntegerOverflow=on
  Out1 : Outport
  wires:
  In1/1 -> Sum2/1
  In2/1 -> Sum2/2
  Sum2/1 -> Sum3/1
  In3/1 -> Sum3/2
  Sum3/1 -> Out1/1

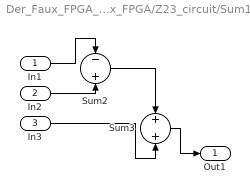
== system Der_Faux_FPGA_V2_optimized_synthesizable/Der_Faux_FPGA/Z23_circuit/Sum1 ==
  In1 : Inport  OutDataTypeStr=fixdt(1,46,42)
  In2 : Inport  Port=2  OutDataTypeStr=fixdt(1,46,54)
  In3 : Inport  Port=3  OutDataTypeStr=fixdt(1,46,54)
  Sum2 : Sum  Inputs=-+  AccumDataTypeStr=fixdt(1,59,54)  OutDataTypeStr=fixdt(1,59,54)  SaturateOnIntegerOverflow=on
  Sum3 : Sum  AccumDataTypeStr=fixdt(1,59,54)  OutDataTypeStr=fixdt(1,46,42)  SaturateOnIntegerOverflow=on
  Out1 : Outport
  wires:
  In1/1 -> Sum2/1
  In2/1 -> Sum2/2
  Sum2/1 -> Sum3/1
  In3/1 -> Sum3/2
  Sum3/1 -> Out1/1

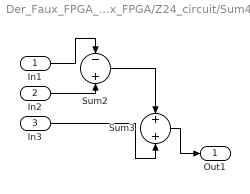
== system Der_Faux_FPGA_V2_optimized_synthesizable/Der_Faux_FPGA/Z24_circuit/Sum4 ==
  In1 : Inport  OutDataTypeStr=fixdt(1,46,43)
  In2 : Inport  Port=2  OutDataTypeStr=fixdt(1,46,54)
  In3 : Inport  Port=3  OutDataTypeStr=fixdt(1,46,54)
  Sum2 : Sum  Inputs=-+  AccumDataTypeStr=fixdt(1,58,54)  OutDataTypeStr=fixdt(1,58,54)  SaturateOnIntegerOverflow=on
  Sum3 : Sum  AccumDataTypeStr=fixdt(1,58,54)  OutDataTypeStr=fixdt(1,46,43)  SaturateOnIntegerOverflow=on
  Out1 : Outport
  wires:
  In1/1 -> Sum2/1
  In2/1 -> Sum2/2
  Sum2/1 -> Sum3/1
  In3/1 -> Sum3/2
  Sum3/1 -> Out1/1

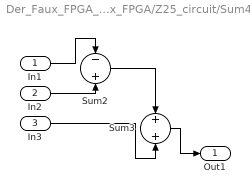
== system Der_Faux_FPGA_V2_optimized_synthesizable/Der_Faux_FPGA/Z25_circuit/Sum4 ==
  In1 : Inport  OutDataTypeStr=fixdt(1,46,42)
  In2 : Inport  Port=2  OutDataTypeStr=fixdt(1,46,50)
  In3 : Inport  Port=3  OutDataTypeStr=fixdt(1,46,50)
  Sum2 : Sum  Inputs=-+  AccumDataTypeStr=fixdt(1,55,50)  OutDataTypeStr=fixdt(1,55,50)  SaturateOnIntegerOverflow=on
  Sum3 : Sum  AccumDataTypeStr=fixdt(1,55,50)  OutDataTypeStr=fixdt(1,46,42)  SaturateOnIntegerOverflow=on
  Out1 : Outport
  wires:
  In1/1 -> Sum2/1
  In2/1 -> Sum2/2
  Sum2/1 -> Sum3/1
  In3/1 -> Sum3/2
  Sum3/1 -> Out1/1
